simulink model "secorderpid2nd"  (R2020a)
settings: Solver=ode23  StartTime=0.0  StopTime=30  FixedStep=1e-3  MaxStep=5e-4  RelTol=5e-4
values from neighbouring files (symbols this model uses):
  b = b+1    (= 2)    [ordenacao.m]
  x0 = nova_populacao(1,:)    [gasearch.m]
undefined symbols (not defined in the file or in its folder): C, d, dx0, K, M
settings Model: SimulationMode=accelerator  Creator=Jose  LastModifiedBy=jhona
settings DataIOCC: LimitDataPoints=on  SaveFormat=Array  SignalLoggingSaveFormat=ModelDataLogs  ReturnWorkspaceOutputs=off
settings OptimizationCC: BlockReduction=off  BooleanDataType=off  ExpressionDepthLimit=2147483647  EfficientMapNaN2IntZero=off  LifeSpan=inf
settings DebuggingCC: SaveWithParameterizedLinksMsg=none  UnderspecifiedInitializationDetection=Classic  MergeDetectMultiDrivingBlocksExec=none  SignalResolutionControl=TryResolveAllWithWarning  MultiTaskDSMMsg=warning  MultiTaskCondExecSysMsg=none  StateNameClashWarn=warning  SFUnexpectedBacktrackingDiag=warning  SFNoUnconditionalDefaultTransitionDiag=warning  SFExecutionAtInitializationDiag=none  ArithmeticOperatorsInVariantConditions=warning
settings HardwareCC: ProdBitPerPointer=32  ProdBitPerSizeT=32  ProdBitPerPtrDiffT=32  ProdLargestAtomicFloat=None  ProdIntDivRoundTo=Undefined  ProdEndianess=Unspecified  ProdWordSize=32  ProdHWDeviceType=32-bit Generic  TargetBitPerPointer=64  TargetBitPerSizeT=64  TargetBitPerPtrDiffT=64  TargetLongLongMode=on  TargetIntDivRoundTo=Zero  TargetEndianess=LittleEndian  TargetWordSize=64  TargetHWDeviceType=MATLAB Host  ProdEqTarget=off
settings ModelReferenceCC: PropagateSignalLabelsOutOfModel=off
settings SFSimCC: SimUseLocalCustomCode=off  CustomCodeUndefinedFunction=UseInterfaceOnly
settings RTWCC: RTWUseLocalCustomCode=off
settings CodeAppCC: MaxIdLength=128  StateflowObjectComments=on
settings GRTTargetCC: TargetLangStandard=C89/C90 (ANSI)  CombineOutputUpdateFcns=off  GRTInterface=on
settings ConfigComp: CovMetricSettings=dw  CovHtmlReporting=on  CovSaveCumulativeToWorkspaceVar=on  CovSaveSingleToWorkspaceVar=on  CovExternalEMLEnable=off

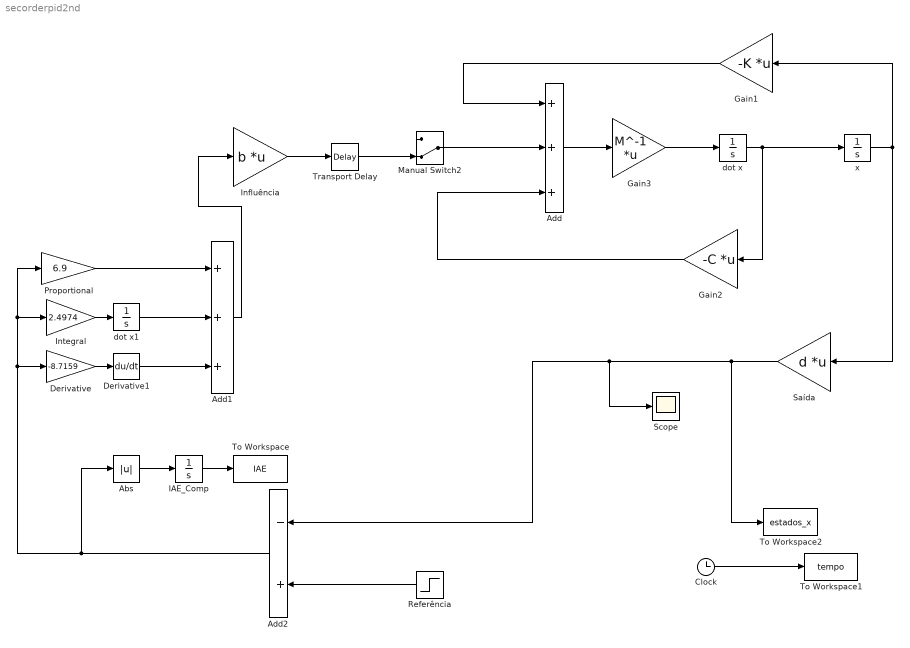
== system secorderpid2nd ==
  Abs : Abs
  Add : Sum  Inputs=+++
  Add1 : Sum  Inputs=+++
  Add2 : Sum  Inputs=-+
  Clock : Clock
  Derivative : Gain  Gain=-8.7159
  Derivative1 : Derivative  CoefficientInTFapproximation=100
  Gain1 : Gain  Gain=-K  Multiplication=Matrix(K*u)
  Gain2 : Gain  Gain=-C  Multiplication=Matrix(K*u)
  Gain3 : Gain  Gain=M^-1  Multiplication=Matrix(K*u)
  IAE_Comp : Integrator
  Influência : Gain  Gain=b  Multiplication=Matrix(K*u)
  Integral : Gain  Gain=2.4974
  Manual Switch2 : ManualSwitch  CurrentSetting=0
  Proportional : Gain  Gain=6.9
  Referência : Step  SampleTime=0
  Saída : Gain  Gain=d  Multiplication=Matrix(K*u)
  Scope : Scope
  To Workspace : ToWorkspace  VariableName=IAE  SampleTime=-1
  To Workspace1 : ToWorkspace  VariableName=tempo  SampleTime=-1
  To Workspace2 : ToWorkspace  VariableName=estados_x  SampleTime=-1
  Transport Delay : TransportDelay  DelayTime=0.1  BufferSize=2048
  dot x : Integrator  InitialCondition=dx0
  dot x1 : Integrator
  x : Integrator  InitialCondition=x0
  wires:
  Gain1/1 -> Add/1
  Add/1 -> Gain3/1
  Gain3/1 -> dot x/1
  dot x/1 -> Gain2/1, x/1
  Gain2/1 -> Add/3
  Influência/1 -> Transport Delay/1
  Manual Switch2/1 -> Add/2
  Transport Delay/1 -> Manual Switch2/2
  Proportional/1 -> Add1/1
  Integral/1 -> dot x1/1
  dot x1/1 -> Add1/2
  Derivative1/1 -> Add1/3
  Derivative/1 -> Derivative1/1
  Referência/1 -> Add2/2
  Add1/1 -> Influência/1
  Add2/1 -> Abs/1, Proportional/1, Integral/1, Derivative/1
  Abs/1 -> IAE_Comp/1
  IAE_Comp/1 -> To Workspace/1
  Clock/1 -> To Workspace1/1
  x/1 -> Saída/1, Gain1/1
  Saída/1 -> To Workspace2/1, Scope/1, Add2/1
